simulink model "BnB"  (Simulink 7.9)
settings: Solver=ode45  StartTime=0.0  StopTime=inf  RelTol=1e-3
values from neighbouring files (symbols this model uses):
  A = [ 0 1  0 0 ; 0 0 m*g/((Ib/r^2) + m) 0 ; 0 0 0 1; -m*g/(Ib + Iball) 0 0 0 ]    [beamandball.m]
  B = [1; 0 ; 0; 1/(Ib+Iball)]    [beamandball.m]
  C = [1 0 0  0]    [beamandball.m]
  K = place(A,B,J)    [beamandball.m]
settings Model: Creator=Prasanth  LastModifiedBy=Prasanth

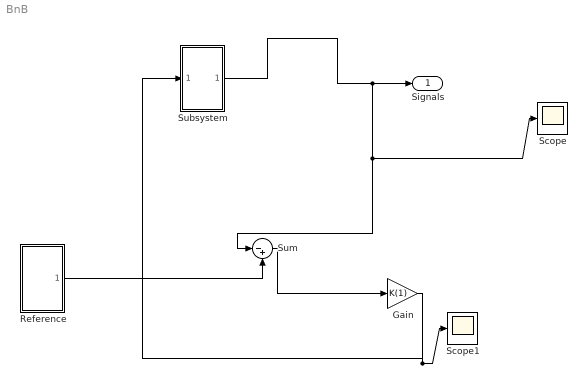
== system BnB ==
  Gain : Gain  Gain=K(1)
  Reference : Subsystem
  Scope : Scope
  Scope1 : Scope
  Subsystem : Subsystem
  Sum : Sum  Inputs=|-+
  Signals : Outport
  wires:
  Subsystem/1(Position) -> Signals/1, Sum/1, Scope/1
  Reference/1(Signals1) -> Sum/2
  Sum/1 -> Gain/1
  Gain/1 -> Subsystem/1(In1), Scope1/1

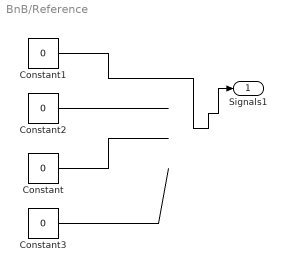
== system BnB/Reference ==
  Constant{,1..3} (4 alike) : Constant  Value=0
  Signals1 : Outport
  wires:
  Constant1/1 -> Signals1/1
  Constant/1 -> ?
  Constant3/1 -> ?
  Constant2/1 -> ?

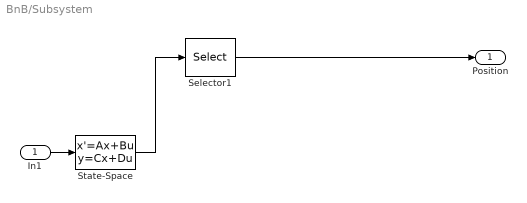
== system BnB/Subsystem ==
  In1 : Inport
  Selector1 : Selector  InputPortWidth=4  IndexOptions=Index vector (dialog)  Indices=1  OutputSizes=1
  State-Space : StateSpace  A=A-B*K  B=B  C=C  D=[ 0; 0;0;0]  X0=[0.1 , 0 , 0, 0]
  Position : Outport
  wires:
  State-Space/1 -> Selector1/1
  Selector1/1 -> Position/1
  In1/1 -> State-Space/1
